simulink model "fuzzy_adaption"  (R2024a)
settings: Solver=VariableStepAuto  StartTime=0.0  StopTime=40  RelTol=1e-3
libraries: fuzblock x2, simulink x1
settings Model: Creator=ericliu  LastModifiedBy=Eason

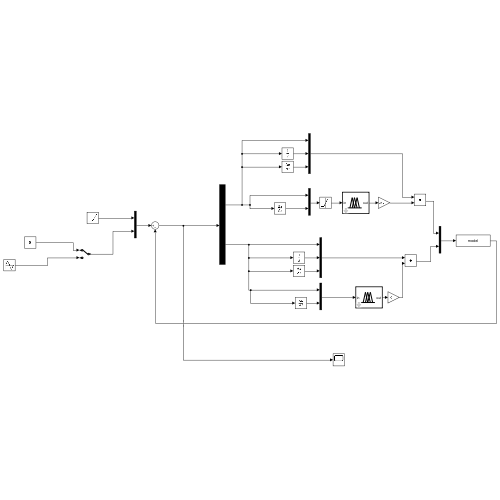
[thumbnail: Simulink's stored preview of the top-level diagram]
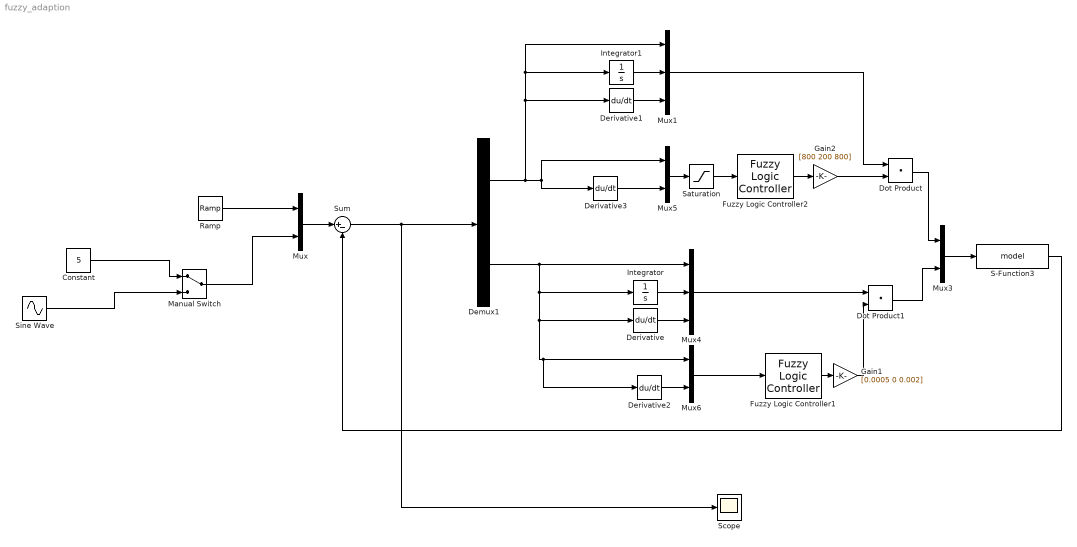
== system fuzzy_adaption ==
  Constant : Constant  Value=5
  Demux1 : Demux  Outputs=2
  Derivative{,1..3} (4 alike) : Derivative
  Dot Product : DotProduct  OutDataTypeStr=Inherit: Inherit via internal rule
  Dot Product1 : DotProduct  OutDataTypeStr=Inherit: Inherit via internal rule
  Fuzzy Logic Controller1 : fuzblock/Fuzzy Logic  Controller  FIS='fuzzyadp.fis'  OutputSampleNumber=101  DataType=double  FuzzifiedInputs=off  RuleFiringStrengths=off  RuleOutputs=off  AggregatedOutputs=off  SimulateUsing=Interpreted execution  OutOfRangeInputValueMessage=warning  NoRuleFiredMessage=warning  EmptyOutputFuzzySetMessage=warning
  Fuzzy Logic Controller2 : fuzblock/Fuzzy Logic  Controller  FIS='fuzzyadp.fis'  OutputSampleNumber=101  DataType=double  FuzzifiedInputs=off  RuleFiringStrengths=off  RuleOutputs=off  AggregatedOutputs=off  SimulateUsing=Interpreted execution  OutOfRangeInputValueMessage=warning  NoRuleFiredMessage=warning  EmptyOutputFuzzySetMessage=warning
  Gain1 : Gain  Gain=[0.0005 0 0.002]
  Gain2 : Gain  Gain=[800 200 800]
  Integrator : Integrator
  Integrator1 : Integrator
  Manual Switch : ManualSwitch
  Mux{,3,5..6} (4 alike) : Mux  Inputs=2
  Mux1 : Mux  Inputs=3
  Mux4 : Mux  Inputs=3
  Ramp : simulink/Sources/Ramp  slope=15  start=0  InitialOutput=0  VectorParams1D=off
  S-Function3 : S-Function  FunctionName=model  SFunctionDeploymentMode=off  EnableBusSupport=off
  Saturation : Saturate  UpperLimit=10  LowerLimit=-10
  Scope : Scope
  Sine Wave : Sin  Amplitude=4  Frequency=0.5  SampleTime=0
  Sum : Sum  Inputs=|+-
  wires:
  Sum/1 -> Scope/1, Demux1/1
  Mux/1 -> Sum/1
  Manual Switch/1 -> Mux/2
  Ramp/1 -> Mux/1
  Demux1/1 -> Mux5/1, Derivative3/1, Mux1/1, Integrator1/1, Derivative1/1
  Demux1/2 -> Mux4/1, Integrator/1, Derivative2/1, Mux6/1, Derivative/1
  Integrator1/1 -> Mux1/2
  Derivative1/1 -> Mux1/3
  S-Function3/1 -> Sum/2
  Derivative3/1 -> Mux5/2
  Integrator/1 -> Mux4/2
  Derivative/1 -> Mux4/3
  Derivative2/1 -> Mux6/2
  Mux1/1 -> Dot Product/1
  Mux5/1 -> Saturation/1
  Dot Product1/1 -> Mux3/2
  Fuzzy Logic Controller2/1 -> Gain2/1
  Fuzzy Logic Controller1/1 -> Gain1/1
  Gain2/1 -> Dot Product/2
  Dot Product/1 -> Mux3/1
  Mux3/1 -> S-Function3/1
  Mux4/1 -> Dot Product1/1
  Gain1/1 -> Dot Product1/2
  Saturation/1 -> Fuzzy Logic Controller2/1
  Mux6/1 -> Fuzzy Logic Controller1/1
  Sine Wave/1 -> Manual Switch/2
  Constant/1 -> Manual Switch/1
